simulink model "Simulation"  (R2022b)
settings: Solver=FixedStepAuto  StartTime=0.0  StopTime=param.Tsim  FixedStep=param.tSample  RelTol=1e-3
StopFcn:
  | run animation
  | run plotSol
undefined symbols (not defined in the file or in its folder): f, filterFr, filterFw, filterMr, FR_neg, FR_pos, g1, g2, g3, kFr, ki, kiSeil, kMr, kp, kpSeil, kVSl, kVSx, MR, MRP, param, xi_0
libraries: simulink x10, spsFirstOrderFilterLib x2
(part 1 of 3)
settings Model: Creator=msdirauf  LastModifiedBy=Khaled
settings SolverCC: AlgebraicLoopSolver=TrustRegion
settings DataIOCC: LimitDataPoints=on  SaveFormat=Array  ReturnWorkspaceOutputs=off
settings OptimizationCC: ExpressionDepthLimit=2147483647  LifeSpan=inf
settings DebuggingCC: UnderspecifiedInitializationDetection=Classic  MergeDetectMultiDrivingBlocksExec=none  SolverPrmCheckMsg=warning  UnconnectedInputMsg=warning  UnconnectedOutputMsg=warning  UnconnectedLineMsg=warning  StateNameClashWarn=warning  SFUnexpectedBacktrackingDiag=warning  SFNoUnconditionalDefaultTransitionDiag=warning  SFExecutionAtInitializationDiag=none  SFMachineParentedDataDiag=warning  ArithmeticOperatorsInVariantConditions=warning
settings HardwareCC: ProdBitPerPointer=32  ProdBitPerSizeT=32  ProdBitPerPtrDiffT=32  ProdLargestAtomicFloat=None  ProdIntDivRoundTo=Undefined  ProdEndianess=Unspecified  ProdWordSize=32  ProdHWDeviceType=32-bit Generic
settings ModelReferenceCC: EnableRefExpFcnMdlSchedulingChecks=on  PropagateSignalLabelsOutOfModel=off
settings SFSimCC: SimUseLocalCustomCode=off  CustomCodeUndefinedFunction=UseInterfaceOnly
settings RTWCC: RTWUseLocalCustomCode=off
settings CodeAppCC: StateflowObjectComments=on
settings GRTTargetCC: TargetLangStandard=C89/C90 (ANSI)
settings ConfigComp: CovMetricSettings=dw  CovSaveCumulativeToWorkspaceVar=on  CovSaveSingleToWorkspaceVar=on  CovExternalEMLEnable=off

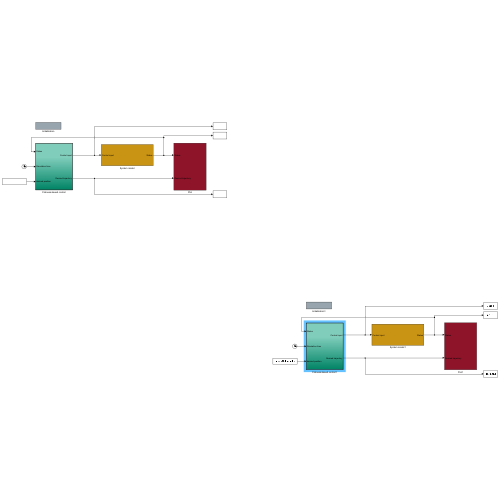
[thumbnail: Simulink's stored preview of the top-level diagram]
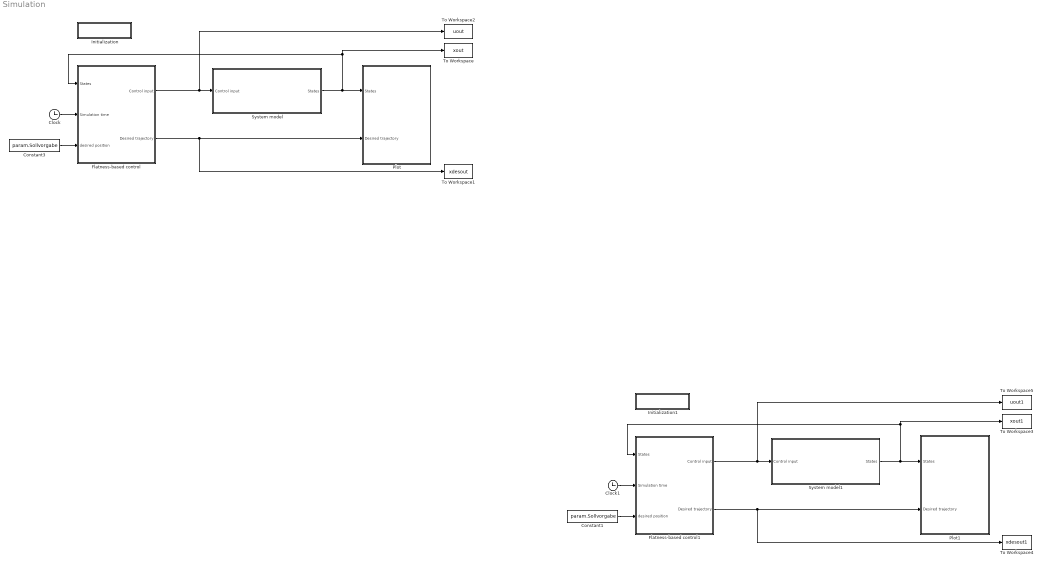
== system Simulation ==
  Clock : Clock
  Clock1 : Clock
  Constant1 : Constant  Value=param.Sollvorgabe
  Constant3 : Constant  Value=param.Sollvorgabe
  Flatness-based control : Subsystem  TreatAsAtomicUnit=on
  Flatness-based control1 : Subsystem  TreatAsAtomicUnit=on
  Initialization : Subsystem
      settings: OpenFcn=run Initialisierung_Simulation
  Initialization1 : Subsystem
      settings: OpenFcn=run Initialisierung_Simulation
  Plot : Subsystem
  Plot1 : Subsystem
  System model : Subsystem
  System model1 : Subsystem
  To Workspace : ToWorkspace  VariableName=xout  SaveFormat=Timeseries  SampleTime=-1
  To Workspace1 : ToWorkspace  VariableName=xdesout  SaveFormat=Timeseries  SampleTime=-1
  To Workspace2 : ToWorkspace  VariableName=uout  SaveFormat=Timeseries  SampleTime=-1
  To Workspace3 : ToWorkspace  VariableName=xout1  SaveFormat=Timeseries  SampleTime=-1
  To Workspace4 : ToWorkspace  VariableName=xdesout1  SaveFormat=Timeseries  SampleTime=-1
  To Workspace5 : ToWorkspace  VariableName=uout1  SaveFormat=Timeseries  SampleTime=-1
  wires:
  Flatness-based control/2(Desired trajectory) -> To Workspace1/1, Plot/2(Desired trajectory)
  Flatness-based control/1(Control input) -> To Workspace2/1, System model/1(Control input)
  Clock/1 -> Flatness-based control/2("Simulation time ")
  Constant3/1 -> Flatness-based control/3(desired position)
  System model/1(States) -> To Workspace/1, Flatness-based control/1(States), Plot/1(States)
  Flatness-based control1/2(Desired trajectory) -> To Workspace4/1, Plot1/2(Desired trajectory)
  Flatness-based control1/1(Control input) -> To Workspace5/1, System model1/1(Control input)
  Clock1/1 -> Flatness-based control1/2("Simulation time ")
  Constant1/1 -> Flatness-based control1/3(desired position)
  System model1/1(States) -> To Workspace3/1, Flatness-based control1/1(States), Plot1/1(States)

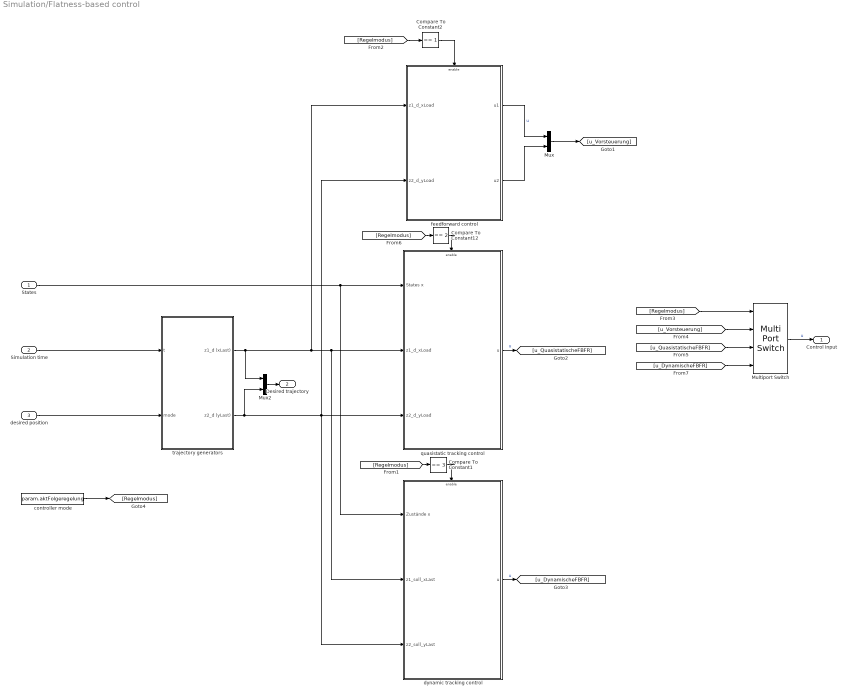
== system Simulation/Flatness-based control ==
  States : Inport
  "Simulation time " : Inport  Port=2
  desired position : Inport  Port=3
  Compare To Constant1 : simulink/Logic and Bit Operations/Compare To Constant  relop===  const=3  OutDataTypeStr=boolean  ZeroCross=off
  Compare To Constant12 : simulink/Logic and Bit Operations/Compare To Constant  relop===  const=2  OutDataTypeStr=boolean  ZeroCross=off
  Compare To Constant2 : simulink/Logic and Bit Operations/Compare To Constant  relop===  const=1  OutDataTypeStr=boolean  ZeroCross=off
  Multiport Switch : MultiPortSwitch  SaturateOnIntegerOverflow=off  InputSameDT=off
  Mux : Mux  Inputs=2
  Mux2 : Mux  Inputs=2
  controller mode : Constant  Value=param.aktFolgeregelung
  dynamic tracking control : Subsystem
  feedforward control : Subsystem
  quasistatic tracking control : Subsystem
  trajectory generators : Subsystem
  Control input : Outport  VectorParamsAs1DForOutWhenUnconnected=off
  Desired trajectory : Outport  Port=2  VectorParamsAs1DForOutWhenUnconnected=off
  wires:
  "Simulation time "/1 -> trajectory generators/1(t)
  trajectory generators/1(z1_d (xLast)) -> Mux2/1, feedforward control/1(z1_d_xLoad), quasistatic tracking control/2(z1_d_xLoad), dynamic tracking control/2(z1_soll_xLast)
  trajectory generators/2(z2_d (yLast)) -> Mux2/2, feedforward control/2(z2_d_yLoad), quasistatic tracking control/3(z2_d_yLoad), dynamic tracking control/3(z2_soll_yLast)
  desired position/1 -> trajectory generators/2(mode)
  Mux2/1 -> Desired trajectory/1
  States/1 -> quasistatic tracking control/1(States x), dynamic tracking control/1(Zustände x)
  Multiport Switch/1 -> Control input/1  "u"
  [Regelmodus] -> Multiport Switch/1
  quasistatic tracking control/1(u) -> [u_QuasistatischeFBFR]  "u"
  [u_QuasistatischeFBFR] -> Multiport Switch/3
  [u_DynamischeFBFR] -> Multiport Switch/4
  [u_Vorsteuerung] -> Multiport Switch/2
  dynamic tracking control/1(u) -> [u_DynamischeFBFR]  "u"
  controller mode/1 -> [Regelmodus]
  Compare To Constant2/1 -> feedforward control/Enable
  [Regelmodus] -> Compare To Constant2/1
  Compare To Constant12/1 -> quasistatic tracking control/Enable
  [Regelmodus] -> Compare To Constant12/1
  [Regelmodus] -> Compare To Constant1/1
  Compare To Constant1/1 -> dynamic tracking control/Enable
  feedforward control/1(u1) -> Mux/1  "u"
  Mux/1 -> [u_Vorsteuerung]
  feedforward control/2(u2) -> Mux/2

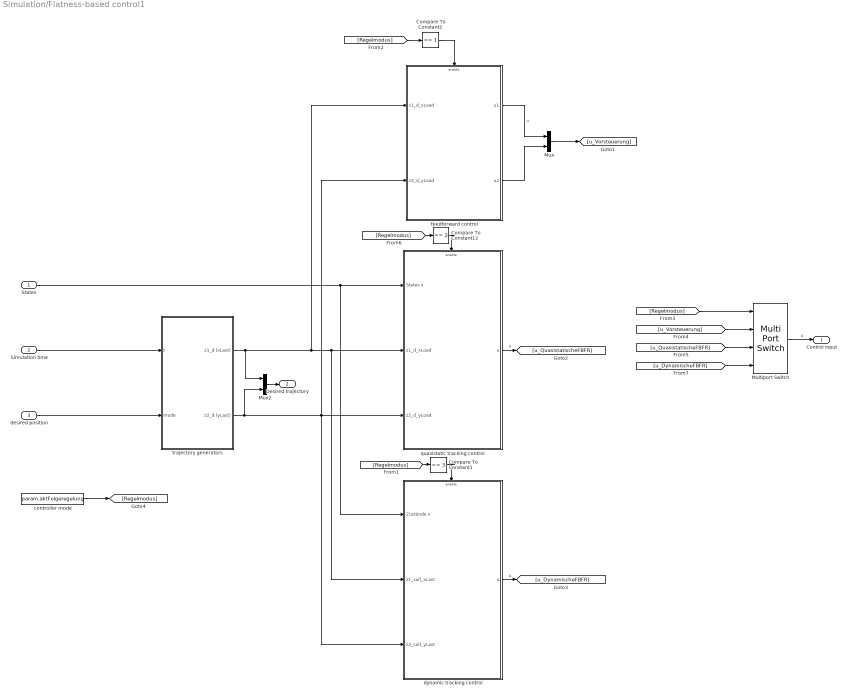
== system Simulation/Flatness-based control1 ==
  States : Inport
  "Simulation time " : Inport  Port=2
  desired position : Inport  Port=3
  Compare To Constant1 : simulink/Logic and Bit Operations/Compare To Constant  relop===  const=3  OutDataTypeStr=boolean  ZeroCross=off
  Compare To Constant12 : simulink/Logic and Bit Operations/Compare To Constant  relop===  const=2  OutDataTypeStr=boolean  ZeroCross=off
  Compare To Constant2 : simulink/Logic and Bit Operations/Compare To Constant  relop===  const=1  OutDataTypeStr=boolean  ZeroCross=off
  Multiport Switch : MultiPortSwitch  SaturateOnIntegerOverflow=off  InputSameDT=off
  Mux : Mux  Inputs=2
  Mux2 : Mux  Inputs=2
  controller mode : Constant  Value=param.aktFolgeregelung
  dynamic tracking control : Subsystem
  feedforward control : Subsystem
  quasistatic tracking control : Subsystem
  trajectory generators : Subsystem
  Control input : Outport  VectorParamsAs1DForOutWhenUnconnected=off
  Desired trajectory : Outport  Port=2  VectorParamsAs1DForOutWhenUnconnected=off
  wires:
  "Simulation time "/1 -> trajectory generators/1(t)
  trajectory generators/1(z1_d (xLast)) -> Mux2/1, feedforward control/1(z1_d_xLoad), quasistatic tracking control/2(z1_d_xLoad), dynamic tracking control/2(z1_soll_xLast)
  trajectory generators/2(z2_d (yLast)) -> Mux2/2, feedforward control/2(z2_d_yLoad), quasistatic tracking control/3(z2_d_yLoad), dynamic tracking control/3(z2_soll_yLast)
  desired position/1 -> trajectory generators/2(mode)
  Mux2/1 -> Desired trajectory/1
  States/1 -> quasistatic tracking control/1(States x), dynamic tracking control/1(Zustände x)
  Multiport Switch/1 -> Control input/1  "u"
  [Regelmodus] -> Multiport Switch/1
  quasistatic tracking control/1(u) -> [u_QuasistatischeFBFR]  "u"
  [u_QuasistatischeFBFR] -> Multiport Switch/3
  [u_DynamischeFBFR] -> Multiport Switch/4
  [u_Vorsteuerung] -> Multiport Switch/2
  dynamic tracking control/1(u) -> [u_DynamischeFBFR]  "u"
  controller mode/1 -> [Regelmodus]
  Compare To Constant2/1 -> feedforward control/Enable
  [Regelmodus] -> Compare To Constant2/1
  Compare To Constant12/1 -> quasistatic tracking control/Enable
  [Regelmodus] -> Compare To Constant12/1
  [Regelmodus] -> Compare To Constant1/1
  Compare To Constant1/1 -> dynamic tracking control/Enable
  feedforward control/1(u1) -> Mux/1  "u"
  Mux/1 -> [u_Vorsteuerung]
  feedforward control/2(u2) -> Mux/2

== system Simulation/Initialization ==

== system Simulation/Initialization1 ==

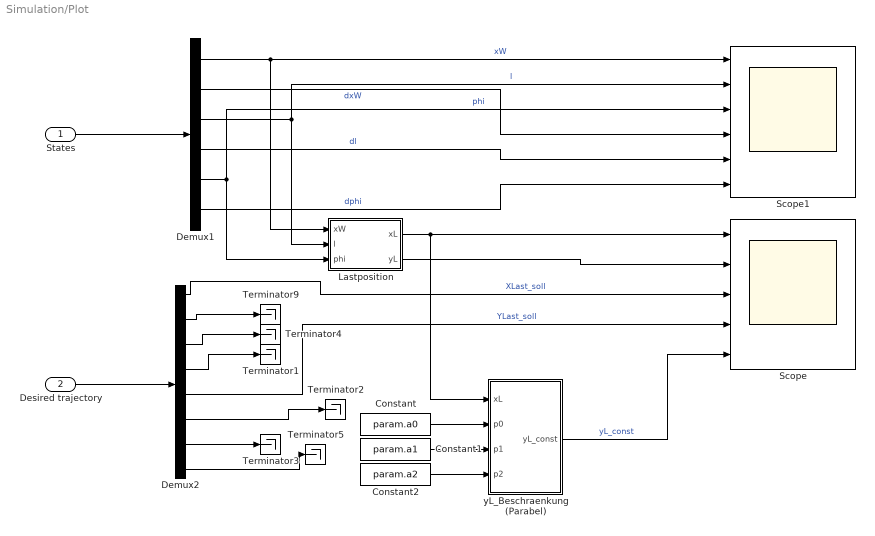
== system Simulation/Plot ==
  States : Inport
  Desired trajectory : Inport  Port=2
  Constant : Constant  Value=param.a0
  Constant1 : Constant  Value=param.a1
  Constant2 : Constant  Value=param.a2
  Demux1 : Demux  Outputs=6
  Demux2 : Demux  Outputs=8
  Lastposition : MATLAB Function  TreatAsAtomicUnit=on
  Scope : Scope  NumInputPorts=5
  Scope1 : Scope  NumInputPorts=6
  Terminator{1..5,9} (6 alike) : Terminator
  yL_Beschraenkung (Parabel) : MATLAB Function  TreatAsAtomicUnit=on
  wires:
  States/1 -> Demux1/1
  Desired trajectory/1 -> Demux2/1
  Demux2/1 -> Scope/3  "XLast_soll"
  Demux2/5 -> Scope/4  "YLast_soll"
  yL_Beschraenkung (Parabel)/1(yL_const) -> Scope/5  "yL_const"
  Demux1/1 -> Lastposition/1(xW), Scope1/1  "xW"
  Lastposition/1(xL) -> yL_Beschraenkung (Parabel)/1(xL), Scope/1
  Lastposition/2(yL) -> Scope/2
  Demux1/3 -> Lastposition/2(l), Scope1/2  "l"
  Demux1/5 -> Lastposition/3(phi), Scope1/3  "phi"
  Demux1/2 -> Scope1/4  "dxW"
  Demux1/4 -> Scope1/5  "dl"
  Demux1/6 -> Scope1/6  "dphi"
  Constant/1 -> yL_Beschraenkung (Parabel)/2(p0)
  Constant1/1 -> yL_Beschraenkung (Parabel)/3(p1)
  Demux2/2 -> Terminator9/1
  Demux2/4 -> Terminator1/1
  Demux2/6 -> Terminator2/1
  Constant2/1 -> yL_Beschraenkung (Parabel)/4(p2)
  Demux2/3 -> Terminator4/1
  Demux2/7 -> Terminator3/1
  Demux2/8 -> Terminator5/1

== system Simulation/Plot1 ==
  States : Inport
  Desired trajectory : Inport  Port=2
  Constant : Constant  Value=param.a0
  Constant1 : Constant  Value=param.a1
  Constant2 : Constant  Value=param.a2
  Demux1 : Demux  Outputs=6
  Demux2 : Demux  Outputs=8
  Lastposition : MATLAB Function  TreatAsAtomicUnit=on
  Scope : Scope  NumInputPorts=5
  Scope1 : Scope  NumInputPorts=6
  Terminator{1..5,9} (6 alike) : Terminator
  yL_Beschraenkung (Parabel) : MATLAB Function  TreatAsAtomicUnit=on
  wires:
  States/1 -> Demux1/1
  Desired trajectory/1 -> Demux2/1
  Demux2/1 -> Scope/3  "XLast_soll"
  Demux2/5 -> Scope/4  "YLast_soll"
  yL_Beschraenkung (Parabel)/1(yL_const) -> Scope/5  "yL_const"
  Demux1/1 -> Lastposition/1(xW), Scope1/1  "xW"
  Lastposition/1(xL) -> yL_Beschraenkung (Parabel)/1(xL), Scope/1
  Lastposition/2(yL) -> Scope/2
  Demux1/3 -> Lastposition/2(l), Scope1/2  "l"
  Demux1/5 -> Lastposition/3(phi), Scope1/3  "phi"
  Demux1/2 -> Scope1/4  "dxW"
  Demux1/4 -> Scope1/5  "dl"
  Demux1/6 -> Scope1/6  "dphi"
  Constant/1 -> yL_Beschraenkung (Parabel)/2(p0)
  Constant1/1 -> yL_Beschraenkung (Parabel)/3(p1)
  Demux2/2 -> Terminator9/1
  Demux2/4 -> Terminator1/1
  Demux2/6 -> Terminator2/1
  Constant2/1 -> yL_Beschraenkung (Parabel)/4(p2)
  Demux2/3 -> Terminator4/1
  Demux2/7 -> Terminator3/1
  Demux2/8 -> Terminator5/1

== system Simulation/System model ==
  Control input : Inport
  Compare To Constant : simulink/Logic and Bit Operations/Compare To Constant  relop===  const=1  OutDataTypeStr=boolean
  Compare To Constant1 : simulink/Logic and Bit Operations/Compare To Constant  relop===  const=0  OutDataTypeStr=boolean
  Constant : Constant  Value=param.Simulationsmodell
  Constant1 : Constant  Value=param.Simulationsmodell
  Constant2 : Constant  Value=param.Simulationsmodell
  Kinematisches Modell : Subsystem
  Referenzmodell : Subsystem  InitFcn=|
      | % Reglerverstaerkungen unterlagerter v-Regler Wagen
      | kp = 25; % 100
      | ki = 0;   % 0 % -> M. Lukassek: Integralanteil nicht nötig, wenn überlagert die flachheitsbasierte Folgeregelung die Sollgrößen adaptiert
      | 
      | % Reglerverstaerkungen unterlagerter v-Regler Seil
      | kpSeil = -20; % -5
      | kiSeil = -0; % -50 -> M. Lukassek: Integralanteil nicht nötig, wenn überlagert die flachheitsbasierte Folgeregelung die Sollgrößen adaptiert
      | 20
      | % Faktor Reibaufschaltung Wagen
      | kFr = 1.0;
      | filterFr = 0.1; % Zeitkonstante der Reibaufschaltung (verhindert hochfreq. Schwingen)
      | 
      | % Faktor Reibaufschaltung Seil
      | kMr = 1.0;
      | filterMr = 0.1; % Zeitkonstante der Reibaufschaltung (verhindert hochfreq. Schwingen)
      |   
      | % Stellgroesse ueberlagerte Regelung verwenden
      | kVSx = 0;  % -> M. Lukassek: Stellgrößen der FBFR als Vorsteuerung für die unterlagerte Regelung. Bypasst die Dead-Band-Reibkompensation
      | kVSl  = 0; % -> M. Lukassek: Stellgrößen der FBFR als Vorsteuerung für die unterlagerte Regelung. Bypasst die Dead-Band-Reibkompensation
      | 
      | % Filterung der Sollkraft Wagen
      | filterFw = 0;
      | filterFwT = 50e-4;
      | 
      | %% Systemparameter
      | g=9.81;
      | 
      | m1=1.43;
      | m2=0.35;
      | J=0.012477;
      | rho=0.03;
      | 
      | muVP=0.0076;
      | F_Tp=0.027;
      | F_Hp=0.012;
      | beta_P=0.073;
      | 
      | muT=0.0097;
      | c_TT=0.6;
      | c_HT=0.41;
      | omega_0=0.015;
      | 
      | mu_W_pos=2.9;
      | c_TW_pos=4.8;
      | c_HW_pos=5.7;
      | v_0_pos=0.032;
      | 
      | mu_W_neg=3.0;
      | c_TW_neg=3.9;
      | c_HW_neg=4.9;
      | v_0_neg=0.022;
      | 
      | muW=0.5*(mu_W_pos+mu_W_neg);
      | 
      | MLast=m2*g*rho;
      | 
      | % Reibparameter des Wagens (positive und negative Bewegungsrichtung)
      | param.mu_W_pos=2.9194;
      | param.c_TW_pos=4.8;
      | param.c_HW_pos=5.7;
      | param.v_0_pos=0.032;
      | 
      | param.mu_W_neg=3.0754;
      | param.c_TW_neg=3.9;
      | param.c_HW_neg=4.9;
      | param.v_0_neg=0.022;
      | 
      | param.muW=0.5*(param.mu_W_pos+param.mu_W_neg);
      | 
      | 
      | % Reibparameter der Trommel
      | param.mu_T=0.0097254;
      | param.c_TT=0.6;
      | param.c_HT=0.41;
      | param.omega_0=0.015;
      | 
      | 
      | param.MLast=param.m2*param.g*param.rho;
      | 
      | % Maximale Antriebskraft des Wagens, maximales Moment des Trommelmotors
      | param.Fmax = 22.5;  
      | param.ScaleFmax = 0.95;
      | 
      | param.M_Tmax = 3.75*rho*13; 
      | 
      | 
      | %Reibmodelle
      | MRP=@(u) u(5)*(muVP*u(2)+F_Tp*sign(u(2))+(F_Hp-F_Tp)*sign(u(2))*exp(-beta_P*abs(u(2))));
      | % ACHTUNG: es ist unklar, ob diese Gleichungen von Hand eingegeben oder
      | % oder automatisch generiert wurden. Falls letzteres, muss in der MAPLE-Quelle
      | % "rho*omega_0" durch "rho/omega_0" ersetzt werden. Hier im Matlabcode
      | % wurde das schon korrigiert.
      | MR=@(u) -(muT*u(6)/rho+c_TT*sign(u(6))+(c_HT-c_TT)*sign(u(6))*exp(-(u(6)/rho/omega_0)^2));
      | FR_pos=@(u) (mu_W_pos*u(4)+c_TW_pos*sign(u(4))+(c_HW_pos-c_TW_pos)*sign(u(4))*exp(-(u(4)/v_0_pos)^2));
      | FR_neg=@(u) (mu_W_neg*u(4)+c_TW_neg*sign(u(4))+(c_HW_neg-c_TW_neg)*sign(u(4))*exp(-(u(4)/v_0_neg)^2));
      | 
      | 
      | %% Maple-Import
      | f=@(u)  [u(2); ((2 * m2 ^ 3 * u(5) * u(2) * u(6) * rho ^ 2) + (2 * m2 ^ 2 * u(5) * u(2) * u(6) * J) + (m2 ^ 3) * g * u(5) * sin(u(1)) * (rho ^ 2) + (m2 ^ 2) * g * u(5) * sin(u(1)) * J - (m2 ^ 3) * g * u(5) * sin(u(1)) ^ 3 * (rho ^ 2) + (m2 ^ 2) * g * u(5) * sin(u(1)) * m1 * (rho ^ 2) + m2 * g * u(5) * sin(u(1)) * m1 * J + (m2 ^ 2) * cos(u(1)) * sin(u(1)) * (u(2) ^ 2) * (u(5) ^ 2) * J - 0.2e1 * (m2 ^ 3) * u(5) * u(2) * u(6) * cos(u(1)) ^ 2 * (rho ^ 2) - 0.2e1 * (m2 ^ 2) * u(5) * u(2) * u(6) * cos(u(1)) ^ 2 * J - 0.2e1 * (m2 ^ 3) * u(5) * u(2) * u(6) * sin(u(1)) ^ 2 * (rho ^ 2) - (m2 ^ 3) * g * u(5) * sin(u(1)) * cos(u(1)) ^ 2 * (rho ^ 2) + 0.2e1 * (m2 ^ 2) * u(5) * u(2) * u(6) * m1 * (rho ^ 2) + 0.2e1 * m2 * u(5) * u(2) * u(6) * m1 * J) / (u(5) ^ 2) / ((m2 ^ 2) * cos(u(1)) ^ 2 * (rho ^ 2) + m2 * cos(u(1)) ^ 2 * J - m1 * m2 * (rho ^ 2) - m1 * J - (m2 ^ 2 * rho ^ 2) - (m2 * J) + (m2 ^ 2) * sin(u(1)) ^ 2 * (rho ^ 2)) / m2; u(4); -0.1e1 / ((m2 ^ 2) * cos(u(1)) ^ 2 * (rho ^ 2) + m2 * cos(u(1)) ^ 2 * J - m1 * m2 * (rho ^ 2) - m1 * J - (m2 ^ 2 * rho ^ 2) - (m2 * J) + (m2 ^ 2) * sin(u(1)) ^ 2 * (rho ^ 2)) * (cos(u(1)) * m2 * g * u(5) * sin(u(1)) * J + m2 * sin(u(1)) * (u(2) ^ 2) * (u(5) ^ 2) * J) / u(5); u(6); ((m2 ^ 2) * sin(u(1)) ^ 2 * rho * cos(u(1)) * g * u(5) - u(5) * m2 * g * cos(u(1)) * rho * m1 - (m2 ^ 2 * u(5) ^ 2 * u(2) ^ 2 * rho) + (m2 ^ 2) * sin(u(1)) ^ 2 * rho * (u(2) ^ 2) * (u(5) ^ 2) + u(5) * (m2 ^ 2) * g * cos(u(1)) ^ 3 * rho - u(5) * (m2 ^ 2) * g * cos(u(1)) * rho + (m2 ^ 2) * (u(5) ^ 2) * (u(2) ^ 2) * rho * cos(u(1)) ^ 2 - m2 * (u(5) ^ 2) * (u(2) ^ 2) * rho * m1) * rho / ((m2 ^ 2) * cos(u(1)) ^ 2 * (rho ^ 2) + m2 * cos(u(1)) ^ 2 * J - m1 * m2 * (rho ^ 2) - m1 * J - (m2 ^ 2 * rho ^ 2) - (m2 * J) + (m2 ^ 2) * sin(u(1)) ^ 2 * (rho ^ 2)) / u(5);];
      | g1=@(u) [0; cos(u(1)) * (m2 * rho ^ 2 + J) / (m2 * cos(u(1)) ^ 2 * J - m2 * J - m1 * m2 * rho ^ 2 - m1 * J) / u(5); 0; -(m2 * rho ^ 2 + J) / (m2 * cos(u(1)) ^ 2 * J - m2 * J - m1 * m2 * rho ^ 2 - m1 * J); 0; m2 * sin(u(1)) * rho ^ 2 / (m2 * cos(u(1)) ^ 2 * J - m2 * J - m1 * m2 * rho ^ 2 - m1 * J);];
      | g2=@(u) [0; m2 * cos(u(1)) * sin(u(1)) * rho / (m2 * cos(u(1)) ^ 2 * J - m2 * J - m1 * m2 * rho ^ 2 - m1 * J) / u(5); 0; -m2 * sin(u(1)) * rho / (m2 * cos(u(1)) ^ 2 * J - m2 * J - m1 * m2 * rho ^ 2 - m1 * J); 0; -rho * (m2 * cos(u(1)) ^ 2 - m1 - m2) / (m2 * cos(u(1)) ^ 2 * J - m2 * J - m1 * m2 * rho ^ 2 - m1 * J);];
      | g3=@(u) [0; (m2 * J + m1 * m2 * rho ^ 2 + m1 * J + m2 ^ 2 * cos(u(1)) ^ 2 * rho ^ 2) / (m2 * cos(u(1)) ^ 2 * J - m2 * J - m1 * m2 * rho ^ 2 - m1 * J) / m2 / u(5) ^ 2; 0; -cos(u(1)) * (m2 * rho ^ 2 + J) / (m2 * cos(u(1)) ^ 2 * J - m2 * J - m1 * m2 * rho ^ 2 - m1 * J) / u(5); 0; m2 * rho ^ 2 * sin(u(1)) * cos(u(1)) / (m2 * cos(u(1)) ^ 2 * J - m2 * J - m1 * m2 * rho ^ 2 - m1 * J) / u(5);];
  Switch : Switch  Criteria=u2 > Threshold  SaturateOnIntegerOverflow=off  InputSameDT=off
  States : Outport  VectorParamsAs1DForOutWhenUnconnected=off
  wires:
  Control input/1 -> Referenzmodell/1(Stellgroessen), Kinematisches Modell/1(Stellgroessen)
  Switch/1 -> States/1
  Kinematisches Modell/1(Systemzustände) -> Switch/3
  Referenzmodell/1(Systemzustaende) -> Switch/1
  Constant/1 -> Switch/2
  Constant1/1 -> Compare To Constant/1
  Compare To Constant/1 -> Referenzmodell/Enable
  Constant2/1 -> Compare To Constant1/1
  Compare To Constant1/1 -> Kinematisches Modell/Enable

== system Simulation/System model1 ==
  Control input : Inport
  Compare To Constant : simulink/Logic and Bit Operations/Compare To Constant  relop===  const=1  OutDataTypeStr=boolean
  Compare To Constant1 : simulink/Logic and Bit Operations/Compare To Constant  relop===  const=0  OutDataTypeStr=boolean
  Constant : Constant  Value=param.Simulationsmodell
  Constant1 : Constant  Value=param.Simulationsmodell
  Constant2 : Constant  Value=param.Simulationsmodell
  Kinematisches Modell : Subsystem
  Referenzmodell : Subsystem  InitFcn=|
      | % Reglerverstaerkungen unterlagerter v-Regler Wagen
      | kp = 25; % 100
      | ki = 0;   % 0 % -> M. Lukassek: Integralanteil nicht nötig, wenn überlagert die flachheitsbasierte Folgeregelung die Sollgrößen adaptiert
      | 
      | % Reglerverstaerkungen unterlagerter v-Regler Seil
      | kpSeil = -20; % -5
      | kiSeil = -0; % -50 -> M. Lukassek: Integralanteil nicht nötig, wenn überlagert die flachheitsbasierte Folgeregelung die Sollgrößen adaptiert
      | 20
      | % Faktor Reibaufschaltung Wagen
      | kFr = 1.0;
      | filterFr = 0.1; % Zeitkonstante der Reibaufschaltung (verhindert hochfreq. Schwingen)
      | 
      | % Faktor Reibaufschaltung Seil
      | kMr = 1.0;
      | filterMr = 0.1; % Zeitkonstante der Reibaufschaltung (verhindert hochfreq. Schwingen)
      |   
      | % Stellgroesse ueberlagerte Regelung verwenden
      | kVSx = 0;  % -> M. Lukassek: Stellgrößen der FBFR als Vorsteuerung für die unterlagerte Regelung. Bypasst die Dead-Band-Reibkompensation
      | kVSl  = 0; % -> M. Lukassek: Stellgrößen der FBFR als Vorsteuerung für die unterlagerte Regelung. Bypasst die Dead-Band-Reibkompensation
      | 
      | % Filterung der Sollkraft Wagen
      | filterFw = 0;
      | filterFwT = 50e-4;
      | 
      | %% Systemparameter
      | g=9.81;
      | 
      | m1=1.43;
      | m2=0.35;
      | J=0.012477;
      | rho=0.03;
      | 
      | muVP=0.0076;
      | F_Tp=0.027;
      | F_Hp=0.012;
      | beta_P=0.073;
      | 
      | muT=0.0097;
      | c_TT=0.6;
      | c_HT=0.41;
      | omega_0=0.015;
      | 
      | mu_W_pos=2.9;
      | c_TW_pos=4.8;
      | c_HW_pos=5.7;
      | v_0_pos=0.032;
      | 
      | mu_W_neg=3.0;
      | c_TW_neg=3.9;
      | c_HW_neg=4.9;
      | v_0_neg=0.022;
      | 
      | muW=0.5*(mu_W_pos+mu_W_neg);
      | 
      | MLast=m2*g*rho;
      | 
      | % Reibparameter des Wagens (positive und negative Bewegungsrichtung)
      | param.mu_W_pos=2.9194;
      | param.c_TW_pos=4.8;
      | param.c_HW_pos=5.7;
      | param.v_0_pos=0.032;
      | 
      | param.mu_W_neg=3.0754;
      | param.c_TW_neg=3.9;
      | param.c_HW_neg=4.9;
      | param.v_0_neg=0.022;
      | 
      | param.muW=0.5*(param.mu_W_pos+param.mu_W_neg);
      | 
      | 
      | % Reibparameter der Trommel
      | param.mu_T=0.0097254;
      | param.c_TT=0.6;
      | param.c_HT=0.41;
      | param.omega_0=0.015;
      | 
      | 
      | param.MLast=param.m2*param.g*param.rho;
      | 
      | % Maximale Antriebskraft des Wagens, maximales Moment des Trommelmotors
      | param.Fmax = 22.5;  
      | param.ScaleFmax = 0.95;
      | 
      | param.M_Tmax = 3.75*rho*13; 
      | 
      | 
      | %Reibmodelle
      | MRP=@(u) u(5)*(muVP*u(2)+F_Tp*sign(u(2))+(F_Hp-F_Tp)*sign(u(2))*exp(-beta_P*abs(u(2))));
      | % ACHTUNG: es ist unklar, ob diese Gleichungen von Hand eingegeben oder
      | % oder automatisch generiert wurden. Falls letzteres, muss in der MAPLE-Quelle
      | % "rho*omega_0" durch "rho/omega_0" ersetzt werden. Hier im Matlabcode
      | % wurde das schon korrigiert.
      | MR=@(u) -(muT*u(6)/rho+c_TT*sign(u(6))+(c_HT-c_TT)*sign(u(6))*exp(-(u(6)/rho/omega_0)^2));
      | FR_pos=@(u) (mu_W_pos*u(4)+c_TW_pos*sign(u(4))+(c_HW_pos-c_TW_pos)*sign(u(4))*exp(-(u(4)/v_0_pos)^2));
      | FR_neg=@(u) (mu_W_neg*u(4)+c_TW_neg*sign(u(4))+(c_HW_neg-c_TW_neg)*sign(u(4))*exp(-(u(4)/v_0_neg)^2));
      | 
      | 
      | %% Maple-Import
      | f=@(u)  [u(2); ((2 * m2 ^ 3 * u(5) * u(2) * u(6) * rho ^ 2) + (2 * m2 ^ 2 * u(5) * u(2) * u(6) * J) + (m2 ^ 3) * g * u(5) * sin(u(1)) * (rho ^ 2) + (m2 ^ 2) * g * u(5) * sin(u(1)) * J - (m2 ^ 3) * g * u(5) * sin(u(1)) ^ 3 * (rho ^ 2) + (m2 ^ 2) * g * u(5) * sin(u(1)) * m1 * (rho ^ 2) + m2 * g * u(5) * sin(u(1)) * m1 * J + (m2 ^ 2) * cos(u(1)) * sin(u(1)) * (u(2) ^ 2) * (u(5) ^ 2) * J - 0.2e1 * (m2 ^ 3) * u(5) * u(2) * u(6) * cos(u(1)) ^ 2 * (rho ^ 2) - 0.2e1 * (m2 ^ 2) * u(5) * u(2) * u(6) * cos(u(1)) ^ 2 * J - 0.2e1 * (m2 ^ 3) * u(5) * u(2) * u(6) * sin(u(1)) ^ 2 * (rho ^ 2) - (m2 ^ 3) * g * u(5) * sin(u(1)) * cos(u(1)) ^ 2 * (rho ^ 2) + 0.2e1 * (m2 ^ 2) * u(5) * u(2) * u(6) * m1 * (rho ^ 2) + 0.2e1 * m2 * u(5) * u(2) * u(6) * m1 * J) / (u(5) ^ 2) / ((m2 ^ 2) * cos(u(1)) ^ 2 * (rho ^ 2) + m2 * cos(u(1)) ^ 2 * J - m1 * m2 * (rho ^ 2) - m1 * J - (m2 ^ 2 * rho ^ 2) - (m2 * J) + (m2 ^ 2) * sin(u(1)) ^ 2 * (rho ^ 2)) / m2; u(4); -0.1e1 / ((m2 ^ 2) * cos(u(1)) ^ 2 * (rho ^ 2) + m2 * cos(u(1)) ^ 2 * J - m1 * m2 * (rho ^ 2) - m1 * J - (m2 ^ 2 * rho ^ 2) - (m2 * J) + (m2 ^ 2) * sin(u(1)) ^ 2 * (rho ^ 2)) * (cos(u(1)) * m2 * g * u(5) * sin(u(1)) * J + m2 * sin(u(1)) * (u(2) ^ 2) * (u(5) ^ 2) * J) / u(5); u(6); ((m2 ^ 2) * sin(u(1)) ^ 2 * rho * cos(u(1)) * g * u(5) - u(5) * m2 * g * cos(u(1)) * rho * m1 - (m2 ^ 2 * u(5) ^ 2 * u(2) ^ 2 * rho) + (m2 ^ 2) * sin(u(1)) ^ 2 * rho * (u(2) ^ 2) * (u(5) ^ 2) + u(5) * (m2 ^ 2) * g * cos(u(1)) ^ 3 * rho - u(5) * (m2 ^ 2) * g * cos(u(1)) * rho + (m2 ^ 2) * (u(5) ^ 2) * (u(2) ^ 2) * rho * cos(u(1)) ^ 2 - m2 * (u(5) ^ 2) * (u(2) ^ 2) * rho * m1) * rho / ((m2 ^ 2) * cos(u(1)) ^ 2 * (rho ^ 2) + m2 * cos(u(1)) ^ 2 * J - m1 * m2 * (rho ^ 2) - m1 * J - (m2 ^ 2 * rho ^ 2) - (m2 * J) + (m2 ^ 2) * sin(u(1)) ^ 2 * (rho ^ 2)) / u(5);];
      | g1=@(u) [0; cos(u(1)) * (m2 * rho ^ 2 + J) / (m2 * cos(u(1)) ^ 2 * J - m2 * J - m1 * m2 * rho ^ 2 - m1 * J) / u(5); 0; -(m2 * rho ^ 2 + J) / (m2 * cos(u(1)) ^ 2 * J - m2 * J - m1 * m2 * rho ^ 2 - m1 * J); 0; m2 * sin(u(1)) * rho ^ 2 / (m2 * cos(u(1)) ^ 2 * J - m2 * J - m1 * m2 * rho ^ 2 - m1 * J);];
      | g2=@(u) [0; m2 * cos(u(1)) * sin(u(1)) * rho / (m2 * cos(u(1)) ^ 2 * J - m2 * J - m1 * m2 * rho ^ 2 - m1 * J) / u(5); 0; -m2 * sin(u(1)) * rho / (m2 * cos(u(1)) ^ 2 * J - m2 * J - m1 * m2 * rho ^ 2 - m1 * J); 0; -rho * (m2 * cos(u(1)) ^ 2 - m1 - m2) / (m2 * cos(u(1)) ^ 2 * J - m2 * J - m1 * m2 * rho ^ 2 - m1 * J);];
      | g3=@(u) [0; (m2 * J + m1 * m2 * rho ^ 2 + m1 * J + m2 ^ 2 * cos(u(1)) ^ 2 * rho ^ 2) / (m2 * cos(u(1)) ^ 2 * J - m2 * J - m1 * m2 * rho ^ 2 - m1 * J) / m2 / u(5) ^ 2; 0; -cos(u(1)) * (m2 * rho ^ 2 + J) / (m2 * cos(u(1)) ^ 2 * J - m2 * J - m1 * m2 * rho ^ 2 - m1 * J) / u(5); 0; m2 * rho ^ 2 * sin(u(1)) * cos(u(1)) / (m2 * cos(u(1)) ^ 2 * J - m2 * J - m1 * m2 * rho ^ 2 - m1 * J) / u(5);];
  Switch : Switch  Criteria=u2 > Threshold  SaturateOnIntegerOverflow=off  InputSameDT=off
  States : Outport  VectorParamsAs1DForOutWhenUnconnected=off
  wires:
  Control input/1 -> Referenzmodell/1(Stellgroessen), Kinematisches Modell/1(Stellgroessen)
  Switch/1 -> States/1
  Kinematisches Modell/1(Systemzustände) -> Switch/3
  Referenzmodell/1(Systemzustaende) -> Switch/1
  Constant/1 -> Switch/2
  Constant1/1 -> Compare To Constant/1
  Compare To Constant/1 -> Referenzmodell/Enable
  Constant2/1 -> Compare To Constant1/1
  Compare To Constant1/1 -> Kinematisches Modell/Enable

== system Simulation/Flatness-based control/dynamic tracking control ==
  Zustände x : Inport
  z1_soll_xLast : Inport  Port=2
  z2_soll_yLast : Inport  Port=3
  EnableDynamischeFBFR : EnablePort  StatesWhenEnabling=reset
  Computation of the flat output : Subsystem
  Mux1 : Mux  Inputs=2
  Mux5 : Mux  Inputs=2
  System extension : Subsystem
  Tracking controller : Subsystem
  Unit Delay1 : UnitDelay  InitialCondition=[0;0]  SampleTime=-1  HasFrameUpgradeWarning=on
  u : Outport
  wires:
  Mux5/1 -> u/1  "u_real"
  System extension/2(x_extended) -> Computation of the flat output/2(States)
  z1_soll_xLast/1 -> Tracking controller/3(z1_d_xLoad)
  Tracking controller/1(u1_aCart) -> Mux5/1, Mux1/1  "u1"
  Computation of the flat output/2(z2_yLoad) -> Tracking controller/2(z2_yLoad)
  Unit Delay1/1 -> System extension/1(u_extended), Computation of the flat output/1(Control input)  "u_old"
  z2_soll_yLast/1 -> Tracking controller/4(z2_d_yLoad)
  Tracking controller/2(u2_aRope) -> Mux1/2  "aRope_d"
  Mux1/1 -> Unit Delay1/1  "u"
  Computation of the flat output/1(z1_xLoad) -> Tracking controller/1(z1_xLoad)
  System extension/1(u2_real) -> Mux5/2  "u2_real"
  Zustände x/1 -> System extension/2(x_real)

== system Simulation/Flatness-based control/feedforward control ==
  z1_d_xLoad : Inport
  z2_d_yLoad : Inport  Port=2
  EnableFBFF : EnablePort  StatesWhenEnabling=reset
  Demux : Demux
  Demux1 : Demux
  MATLAB Function : MATLAB Function  TreatAsAtomicUnit=on
  u1 : Outport
  u2 : Outport  Port=2
  wires:
  z1_d_xLoad/1 -> Demux/1
  MATLAB Function/1(u1) -> u1/1
  MATLAB Function/2(u2) -> u2/1
  Demux/1 -> MATLAB Function/1(z1)
  Demux/2 -> MATLAB Function/2(dz1)
  Demux/3 -> MATLAB Function/3(ddz1)
  z2_d_yLoad/1 -> Demux1/1
  Demux1/1 -> MATLAB Function/5(z2)
  Demux1/2 -> MATLAB Function/6(dz2)
  Demux1/3 -> MATLAB Function/7(ddz2)
  Demux/4 -> MATLAB Function/4(d3z1)
  Demux1/4 -> MATLAB Function/8(d3z2)

== system Simulation/Flatness-based control/quasistatic tracking control ==
  States x : Inport
  z1_d_xLoad : Inport  Port=2
  z2_d_yLoad : Inport  Port=3
  EnableQuasistatischeFBFR : EnablePort  StatesWhenEnabling=reset
  Computation of the flat output : Subsystem
  Mux : Mux  Inputs=2
  Tracking controller : Subsystem
  Unit Delay : UnitDelay  InitialCondition=[0;0]  SampleTime=-1  HasFrameUpgradeWarning=on
  u : Outport
  wires:
  Computation of the flat output/2(z2_yLoad) -> Tracking controller/2(z2_yLoad)
  Computation of the flat output/1(z1_xLoad) -> Tracking controller/1(z1_xLoad)
  Tracking controller/2(u2_aRope) -> Mux/2  "aRope_d"
  Mux/1 -> u/1, Unit Delay/1  "u"
  Unit Delay/1 -> Computation of the flat output/1(Control input)  "u_old"
  States x/1 -> Computation of the flat output/2(States)
  Tracking controller/1(u1_aCart) -> Mux/1  "u1"
  z1_d_xLoad/1 -> Tracking controller/3(z1_d_xLoad)
  z2_d_yLoad/1 -> Tracking controller/4(z2_d_yLoad)

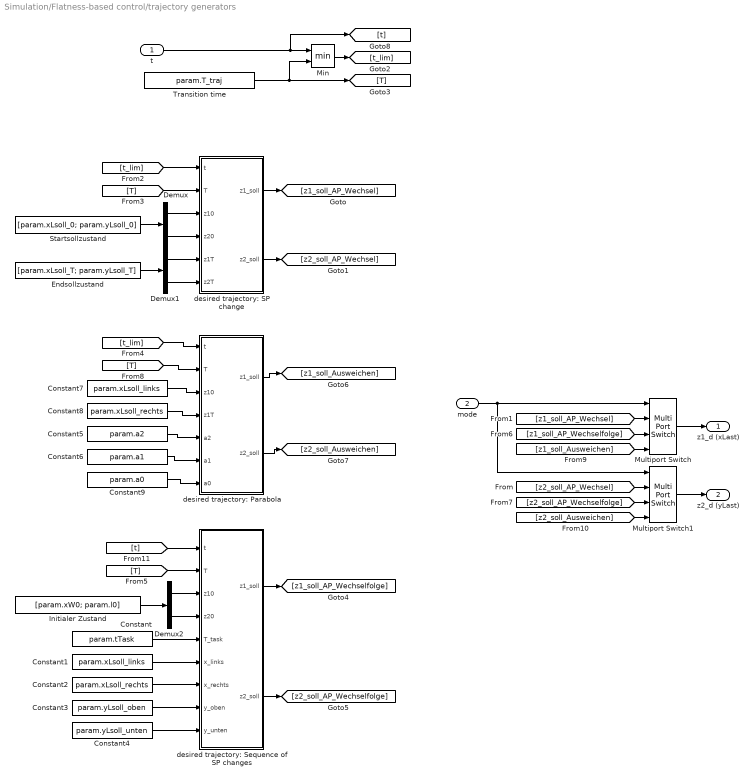
== system Simulation/Flatness-based control/trajectory generators ==
  t : Inport
  mode : Inport  Port=2
  Constant : Constant  Value=param.tTask
  Constant1 : Constant  Value=param.xLsoll_links
  Constant2 : Constant  Value=param.xLsoll_rechts
  Constant3 : Constant  Value=param.yLsoll_oben
  Constant4 : Constant  Value=param.yLsoll_unten
  Constant5 : Constant  Value=param.a2
  Constant6 : Constant  Value=param.a1
  Constant7 : Constant  Value=param.xLsoll_links
  Constant8 : Constant  Value=param.xLsoll_rechts
  Constant9 : Constant  Value=param.a0
  Demux : Demux  Outputs=2
  Demux1 : Demux  Outputs=2
  Demux2 : Demux  Outputs=2
  Endsollzustand : Constant  Value=[param.xLsoll_T; param.yLsoll_T]
  Initialer Zustand : Constant  Value=[param.xW0; param.l0]
  Min : MinMax  Inputs=2
  Multiport Switch : MultiPortSwitch  SaturateOnIntegerOverflow=off  InputSameDT=off
  Multiport Switch1 : MultiPortSwitch  SaturateOnIntegerOverflow=off  InputSameDT=off
  Startsollzustand : Constant  Value=[param.xLsoll_0; param.yLsoll_0]
  Transition time : Constant  Value=param.T_traj
  desired trajectory: Parabola : MATLAB Function  TreatAsAtomicUnit=on
  desired trajectory: SP change : MATLAB Function  TreatAsAtomicUnit=on
  desired trajectory: Sequence of SP changes : MATLAB Function  TreatAsAtomicUnit=on
  z1_d (xLast) : Outport
  z2_d (yLast) : Outport  Port=2
  wires:
  Transition time/1 -> [T], Min/2
  mode/1 -> Multiport Switch/1, Multiport Switch1/1
  Multiport Switch1/1 -> z2_d (yLast)/1
  Multiport Switch/1 -> z1_d (xLast)/1
  [z2_soll_AP_Wechsel] -> Multiport Switch1/2
  [z1_soll_AP_Wechsel] -> Multiport Switch/2
  Min/1 -> [t_lim]
  t/1 -> [t], Min/1
  [z1_soll_AP_Wechselfolge] -> Multiport Switch/3
  [z2_soll_AP_Wechselfolge] -> Multiport Switch1/3
  Startsollzustand/1 -> Demux/1
  Endsollzustand/1 -> Demux1/1
  [z1_soll_Ausweichen] -> Multiport Switch/4
  [z2_soll_Ausweichen] -> Multiport Switch1/4
  Initialer Zustand/1 -> Demux2/1
  [t_lim] -> desired trajectory: SP change/1(t)
  [T] -> desired trajectory: SP change/2(T)
  Demux/1 -> desired trajectory: SP change/3(z10)
  Demux/2 -> desired trajectory: SP change/4(z20)
  Demux1/1 -> desired trajectory: SP change/5(z1T)
  Demux1/2 -> desired trajectory: SP change/6(z2T)
  desired trajectory: SP change/1(z1_soll) -> [z1_soll_AP_Wechsel]
  desired trajectory: SP change/2(z2_soll) -> [z2_soll_AP_Wechsel]
  [t_lim] -> desired trajectory: Parabola/1(t)
  [T] -> desired trajectory: Parabola/2(T)
  Constant7/1 -> desired trajectory: Parabola/3(z10)
  Constant8/1 -> desired trajectory: Parabola/4(z1T)
  Constant5/1 -> desired trajectory: Parabola/5(a2)
  Constant6/1 -> desired trajectory: Parabola/6(a1)
  Constant9/1 -> desired trajectory: Parabola/7(a0)
  desired trajectory: Parabola/1(z1_soll) -> [z1_soll_Ausweichen]
  desired trajectory: Parabola/2(z2_soll) -> [z2_soll_Ausweichen]
  [t] -> desired trajectory: Sequence of SP changes/1(t)
  [T] -> desired trajectory: Sequence of SP changes/2(T)
  Demux2/1 -> desired trajectory: Sequence of SP changes/3(z10)
  Demux2/2 -> desired trajectory: Sequence of SP changes/4(z20)
  Constant/1 -> desired trajectory: Sequence of SP changes/5(T_task)
  Constant1/1 -> desired trajectory: Sequence of SP changes/6(x_links)
  Constant2/1 -> desired trajectory: Sequence of SP changes/7(x_rechts)
  Constant3/1 -> desired trajectory: Sequence of SP changes/8(y_oben)
  Constant4/1 -> desired trajectory: Sequence of SP changes/9(y_unten)
  desired trajectory: Sequence of SP changes/1(z1_soll) -> [z1_soll_AP_Wechselfolge]
  desired trajectory: Sequence of SP changes/2(z2_soll) -> [z2_soll_AP_Wechselfolge]

== system Simulation/Flatness-based control1/dynamic tracking control ==
  Zustände x : Inport
  z1_soll_xLast : Inport  Port=2
  z2_soll_yLast : Inport  Port=3
  EnableDynamischeFBFR : EnablePort  StatesWhenEnabling=reset
  Computation of the flat output : Subsystem
  Mux1 : Mux  Inputs=2
  Mux5 : Mux  Inputs=2
  System extension : Subsystem
  Tracking controller : Subsystem
  Unit Delay1 : UnitDelay  InitialCondition=[0;0]  SampleTime=-1  HasFrameUpgradeWarning=on
  u : Outport
  wires:
  Mux5/1 -> u/1  "u_real"
  System extension/2(x_extended) -> Computation of the flat output/2(States)
  z1_soll_xLast/1 -> Tracking controller/3(z1_d_xLoad)
  Tracking controller/1(u1_aCart) -> Mux5/1, Mux1/1  "u1"
  Computation of the flat output/2(z2_yLoad) -> Tracking controller/2(z2_yLoad)
  Unit Delay1/1 -> System extension/1(u_extended), Computation of the flat output/1(Control input)  "u_old"
  z2_soll_yLast/1 -> Tracking controller/4(z2_d_yLoad)
  Tracking controller/2(u2_aRope) -> Mux1/2  "aRope_d"
  Mux1/1 -> Unit Delay1/1  "u"
  Computation of the flat output/1(z1_xLoad) -> Tracking controller/1(z1_xLoad)
  System extension/1(u2_real) -> Mux5/2  "u2_real"
  Zustände x/1 -> System extension/2(x_real)

== system Simulation/Flatness-based control1/feedforward control ==
  z1_d_xLoad : Inport
  z2_d_yLoad : Inport  Port=2
  EnableFBFF : EnablePort  StatesWhenEnabling=reset
  Demux : Demux
  Demux1 : Demux
  MATLAB Function : MATLAB Function  TreatAsAtomicUnit=on
  u1 : Outport
  u2 : Outport  Port=2
  wires:
  z1_d_xLoad/1 -> Demux/1
  MATLAB Function/1(u1) -> u1/1
  MATLAB Function/2(u2) -> u2/1
  Demux/1 -> MATLAB Function/1(z1)
  Demux/2 -> MATLAB Function/2(dz1)
  Demux/3 -> MATLAB Function/3(ddz1)
  z2_d_yLoad/1 -> Demux1/1
  Demux1/1 -> MATLAB Function/5(z2)
  Demux1/2 -> MATLAB Function/6(dz2)
  Demux1/3 -> MATLAB Function/7(ddz2)
  Demux/4 -> MATLAB Function/4(d3z1)
  Demux1/4 -> MATLAB Function/8(d3z2)

== system Simulation/Flatness-based control1/quasistatic tracking control ==
  States x : Inport
  z1_d_xLoad : Inport  Port=2
  z2_d_yLoad : Inport  Port=3
  EnableQuasistatischeFBFR : EnablePort  StatesWhenEnabling=reset
  Computation of the flat output : Subsystem
  Mux : Mux  Inputs=2
  Tracking controller : Subsystem
  Unit Delay : UnitDelay  InitialCondition=[0;0]  SampleTime=-1  HasFrameUpgradeWarning=on
  u : Outport
  wires:
  Computation of the flat output/2(z2_yLoad) -> Tracking controller/2(z2_yLoad)
  Computation of the flat output/1(z1_xLoad) -> Tracking controller/1(z1_xLoad)
  Tracking controller/2(u2_aRope) -> Mux/2  "aRope_d"
  Mux/1 -> u/1, Unit Delay/1  "u"
  Unit Delay/1 -> Computation of the flat output/1(Control input)  "u_old"
  States x/1 -> Computation of the flat output/2(States)
  Tracking controller/1(u1_aCart) -> Mux/1  "u1"
  z1_d_xLoad/1 -> Tracking controller/3(z1_d_xLoad)
  z2_d_yLoad/1 -> Tracking controller/4(z2_d_yLoad)

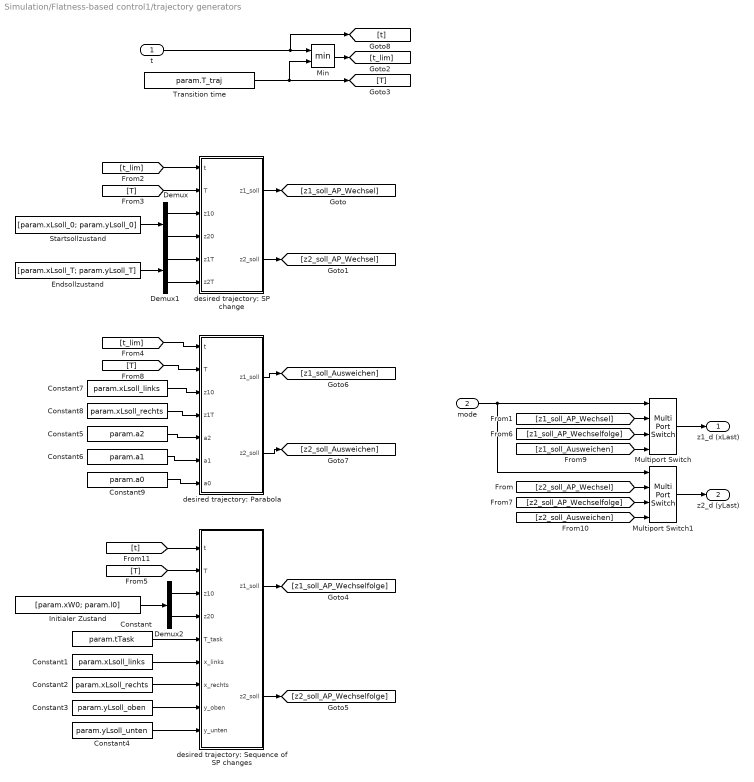
== system Simulation/Flatness-based control1/trajectory generators ==
  t : Inport
  mode : Inport  Port=2
  Constant : Constant  Value=param.tTask
  Constant1 : Constant  Value=param.xLsoll_links
  Constant2 : Constant  Value=param.xLsoll_rechts
  Constant3 : Constant  Value=param.yLsoll_oben
  Constant4 : Constant  Value=param.yLsoll_unten
  Constant5 : Constant  Value=param.a2
  Constant6 : Constant  Value=param.a1
  Constant7 : Constant  Value=param.xLsoll_links
  Constant8 : Constant  Value=param.xLsoll_rechts
  Constant9 : Constant  Value=param.a0
  Demux : Demux  Outputs=2
  Demux1 : Demux  Outputs=2
  Demux2 : Demux  Outputs=2
  Endsollzustand : Constant  Value=[param.xLsoll_T; param.yLsoll_T]
  Initialer Zustand : Constant  Value=[param.xW0; param.l0]
  Min : MinMax  Inputs=2
  Multiport Switch : MultiPortSwitch  SaturateOnIntegerOverflow=off  InputSameDT=off
  Multiport Switch1 : MultiPortSwitch  SaturateOnIntegerOverflow=off  InputSameDT=off
  Startsollzustand : Constant  Value=[param.xLsoll_0; param.yLsoll_0]
  Transition time : Constant  Value=param.T_traj
  desired trajectory: Parabola : MATLAB Function  TreatAsAtomicUnit=on
  desired trajectory: SP change : MATLAB Function  TreatAsAtomicUnit=on
  desired trajectory: Sequence of SP changes : MATLAB Function  TreatAsAtomicUnit=on
  z1_d (xLast) : Outport
  z2_d (yLast) : Outport  Port=2
  wires:
  Transition time/1 -> [T], Min/2
  mode/1 -> Multiport Switch/1, Multiport Switch1/1
  Multiport Switch1/1 -> z2_d (yLast)/1
  Multiport Switch/1 -> z1_d (xLast)/1
  [z2_soll_AP_Wechsel] -> Multiport Switch1/2
  [z1_soll_AP_Wechsel] -> Multiport Switch/2
  Min/1 -> [t_lim]
  t/1 -> [t], Min/1
  [z1_soll_AP_Wechselfolge] -> Multiport Switch/3
  [z2_soll_AP_Wechselfolge] -> Multiport Switch1/3
  Startsollzustand/1 -> Demux/1
  Endsollzustand/1 -> Demux1/1
  [z1_soll_Ausweichen] -> Multiport Switch/4
  [z2_soll_Ausweichen] -> Multiport Switch1/4
  Initialer Zustand/1 -> Demux2/1
  [t_lim] -> desired trajectory: SP change/1(t)
  [T] -> desired trajectory: SP change/2(T)
  Demux/1 -> desired trajectory: SP change/3(z10)
  Demux/2 -> desired trajectory: SP change/4(z20)
  Demux1/1 -> desired trajectory: SP change/5(z1T)
  Demux1/2 -> desired trajectory: SP change/6(z2T)
  desired trajectory: SP change/1(z1_soll) -> [z1_soll_AP_Wechsel]
  desired trajectory: SP change/2(z2_soll) -> [z2_soll_AP_Wechsel]
  [t_lim] -> desired trajectory: Parabola/1(t)
  [T] -> desired trajectory: Parabola/2(T)
  Constant7/1 -> desired trajectory: Parabola/3(z10)
  Constant8/1 -> desired trajectory: Parabola/4(z1T)
  Constant5/1 -> desired trajectory: Parabola/5(a2)
  Constant6/1 -> desired trajectory: Parabola/6(a1)
  Constant9/1 -> desired trajectory: Parabola/7(a0)
  desired trajectory: Parabola/1(z1_soll) -> [z1_soll_Ausweichen]
  desired trajectory: Parabola/2(z2_soll) -> [z2_soll_Ausweichen]
  [t] -> desired trajectory: Sequence of SP changes/1(t)
  [T] -> desired trajectory: Sequence of SP changes/2(T)
  Demux2/1 -> desired trajectory: Sequence of SP changes/3(z10)
  Demux2/2 -> desired trajectory: Sequence of SP changes/4(z20)
  Constant/1 -> desired trajectory: Sequence of SP changes/5(T_task)
  Constant1/1 -> desired trajectory: Sequence of SP changes/6(x_links)
  Constant2/1 -> desired trajectory: Sequence of SP changes/7(x_rechts)
  Constant3/1 -> desired trajectory: Sequence of SP changes/8(y_oben)
  Constant4/1 -> desired trajectory: Sequence of SP changes/9(y_unten)
  desired trajectory: Sequence of SP changes/1(z1_soll) -> [z1_soll_AP_Wechselfolge]
  desired trajectory: Sequence of SP changes/2(z2_soll) -> [z2_soll_AP_Wechselfolge]

== system Simulation/System model/Kinematisches Modell ==
  Stellgroessen : Inport
  Enable : EnablePort
  Integrator : Integrator  InitialCondition=[param.xW0, 0.0, param.l0, 0.0, 0.0, 0.0]
  "sys_dgl " : MATLAB Function  TreatAsAtomicUnit=on
  Systemzustände : Outport
  wires:
  "sys_dgl "/1(dx) -> Integrator/1
  Integrator/1 -> Systemzustände/1, "sys_dgl "/1(x)
  Stellgroessen/1 -> "sys_dgl "/2(u)

== system Simulation/System model/Referenzmodell ==
  Stellgroessen : Inport
  Enable : EnablePort
  Constant5 : Constant  Value=[0 0 param.xW0 0 param.l0 0]
  Demux : Demux  Outputs=2
  Integrator : Integrator
  Integrator1 : Integrator
  Referenzstrecke : Subsystem
  Selector : Selector  InputPortWidth=6  IndexOptions=Index vector (dialog)  Indices=4  OutputSizes=1
  Selector1 : Selector  InputPortWidth=6  IndexOptions=Index vector (dialog)  Indices=6  OutputSizes=1
  Unterlagerte v-Regelung : Subsystem
  Vorsteuerung Trommel : Subsystem
  Vorsteuerung Wagen : Subsystem
  Zustandsvektor : Selector  InputPortWidth=6  IndexOptions=Index vector (dialog)  Indices=[3 4 5 6 1 2]  OutputSizes=1
  Systemzustaende : Outport
  wires:
  Selector/1 -> Unterlagerte v-Regelung/1(vW)  "vW"
  Selector1/1 -> Unterlagerte v-Regelung/2(vl)  "vL"
  Constant5/1 -> Referenzstrecke/2(xi0)
  Referenzstrecke/1("xi (phi, phip, x, xp, l, lp)") -> Selector/1, Selector1/1, Zustandsvektor/1  "x_truth"
  Zustandsvektor/1 -> Systemzustaende/1  "5"
  Unterlagerte v-Regelung/1(u) -> Referenzstrecke/1("u (F, MT)")
  Stellgroessen/1 -> Demux/1
  Integrator/1 -> Unterlagerte v-Regelung/3(vWDes)
  Integrator1/1 -> Unterlagerte v-Regelung/4(vldes)
  Demux/1 -> Integrator/1, Vorsteuerung Wagen/1(aW)
  Demux/2 -> Vorsteuerung Trommel/1(aS), Integrator1/1
  Vorsteuerung Trommel/1(FF MT) -> Unterlagerte v-Regelung/6(FW_MT)
  Vorsteuerung Wagen/1(FF FW) -> Unterlagerte v-Regelung/5(FW_VS)

== system Simulation/System model1/Kinematisches Modell ==
  Stellgroessen : Inport
  Enable : EnablePort
  Integrator : Integrator  InitialCondition=[param.xW0, 0.0, param.l0, 0.0, 0.0, 0.0]
  "sys_dgl " : MATLAB Function  TreatAsAtomicUnit=on
  Systemzustände : Outport
  wires:
  "sys_dgl "/1(dx) -> Integrator/1
  Integrator/1 -> Systemzustände/1, "sys_dgl "/1(x)
  Stellgroessen/1 -> "sys_dgl "/2(u)

== system Simulation/System model1/Referenzmodell ==
  Stellgroessen : Inport
  Enable : EnablePort
  Constant5 : Constant  Value=[0 0 param.xW0 0 param.l0 0]
  Demux : Demux  Outputs=2
  Integrator : Integrator
  Integrator1 : Integrator
  Referenzstrecke : Subsystem
  Selector : Selector  InputPortWidth=6  IndexOptions=Index vector (dialog)  Indices=4  OutputSizes=1
  Selector1 : Selector  InputPortWidth=6  IndexOptions=Index vector (dialog)  Indices=6  OutputSizes=1
  Unterlagerte v-Regelung : Subsystem
  Vorsteuerung Trommel : Subsystem
  Vorsteuerung Wagen : Subsystem
  Zustandsvektor : Selector  InputPortWidth=6  IndexOptions=Index vector (dialog)  Indices=[3 4 5 6 1 2]  OutputSizes=1
  Systemzustaende : Outport
  wires:
  Selector/1 -> Unterlagerte v-Regelung/1(vW)  "vW"
  Selector1/1 -> Unterlagerte v-Regelung/2(vl)  "vL"
  Constant5/1 -> Referenzstrecke/2(xi0)
  Referenzstrecke/1("xi (phi, phip, x, xp, l, lp)") -> Selector/1, Selector1/1, Zustandsvektor/1  "x_truth"
  Zustandsvektor/1 -> Systemzustaende/1  "5"
  Unterlagerte v-Regelung/1(u) -> Referenzstrecke/1("u (F, MT)")
  Stellgroessen/1 -> Demux/1
  Integrator/1 -> Unterlagerte v-Regelung/3(vWDes)
  Integrator1/1 -> Unterlagerte v-Regelung/4(vldes)
  Demux/1 -> Integrator/1, Vorsteuerung Wagen/1(aW)
  Demux/2 -> Vorsteuerung Trommel/1(aS), Integrator1/1
  Vorsteuerung Trommel/1(FF MT) -> Unterlagerte v-Regelung/6(FW_MT)
  Vorsteuerung Wagen/1(FF FW) -> Unterlagerte v-Regelung/5(FW_VS)

== system Simulation/Flatness-based control/dynamic tracking control/Computation of the flat output ==
  Control input : Inport
  States : Inport  Port=2
  Demux : Demux  Outputs=8
  Demux1 : Demux  Outputs=2
  Derivative : Derivative
  Derivative1 : Derivative
  MATLAB Function : MATLAB Function  TreatAsAtomicUnit=on
  MATLAB Function1 : MATLAB Function  TreatAsAtomicUnit=on
  MATLAB Function2 : MATLAB Function  TreatAsAtomicUnit=on
  Mux : Mux
  Mux1 : Mux
  z1_xLoad : Outport
  z2_yLoad : Outport  Port=2
  wires:
  MATLAB Function/2(z2) -> Mux1/1
  Derivative/1 -> Mux/4
  MATLAB Function2/1(ddz1) -> Mux/3, Derivative/1
  MATLAB Function/1(z1) -> Mux/1
  Demux/2 -> MATLAB Function1/1(x2)
  Demux/6 -> MATLAB Function2/3(x6), MATLAB Function1/5(x6)
  MATLAB Function2/2(ddz2) -> Mux1/3, Derivative1/1
  Control input/1 -> Demux1/1
  MATLAB Function1/2(dz2) -> Mux1/2
  Demux/5 -> MATLAB Function/3(x5), MATLAB Function2/2(x5), MATLAB Function1/4(x5)
  Demux/1 -> MATLAB Function/1(x1)
  States/1 -> Demux/1
  Demux/3 -> MATLAB Function2/1(x3), MATLAB Function1/2(x3), MATLAB Function/2(x3)
  Demux/4 -> MATLAB Function1/3(x4)
  MATLAB Function1/1(dz1) -> Mux/2
  Derivative1/1 -> Mux1/4
  Mux/1 -> z1_xLoad/1
  Mux1/1 -> z2_yLoad/1
  Demux1/1 -> MATLAB Function2/4(u1)
  Demux1/2 -> MATLAB Function2/5(u2)

== system Simulation/Flatness-based control/dynamic tracking control/System extension ==
  u_extended : Inport
  x_real : Inport  Port=2
  Demux : Demux  Outputs=6
  Demux1 : Demux  Outputs=2
  Integrator : Integrator
  Integrator1 : Integrator
  MATLAB Function3 : MATLAB Function  TreatAsAtomicUnit=on
  Mux : Mux  Inputs=8
  u2_real : Outport
  x_extended : Outport  Port=2
  wires:
  u_extended/1 -> Demux1/1
  x_real/1 -> Demux/1
  Mux/1 -> x_extended/1
  Demux/1 -> Mux/1
  Demux1/1 -> MATLAB Function3/5(u1_ext), Mux/2
  Demux/3 -> Mux/3, MATLAB Function3/2(x3)
  MATLAB Function3/1(u2_real) -> Mux/4, u2_real/1
  Demux/5 -> MATLAB Function3/3(x5), Mux/5
  Demux/6 -> Mux/6, MATLAB Function3/4(x6)
  Demux1/2 -> Integrator/1
  Integrator/1 -> Mux/8, Integrator1/1  "x2_ext"
  Integrator1/1 -> Mux/7, MATLAB Function3/1(x1_ext)  "x1_ext"

== system Simulation/Flatness-based control/dynamic tracking control/Tracking controller ==
  z1_xLoad : Inport
  z2_yLoad : Inport  Port=2
  z1_d_xLoad : Inport  Port=3
  z2_d_yLoad : Inport  Port=4
  Constant : Constant  Value=[param.pX01 param.pX02 param.pX03 param.pX04]
  Constant1 : Constant  Value=[param.pY01_DYN param.pY02_DYN param.pY03_DYN param.pY04_DYN]
  Demux : Demux
  Demux1 : Demux
  MATLAB Function : MATLAB Function  TreatAsAtomicUnit=on
  Tracking controller v1 for xLoad : Subsystem
  Tracking controller v2 for yLoad : Subsystem
  u1_aCart : Outport
  u2_aRope : Outport  Port=2
  wires:
  Constant1/1 -> Tracking controller v2 for yLoad/3(Koeffizienten2)
  Constant/1 -> Tracking controller v1 for xLoad/3(Koeffizienten1)
  z2_d_yLoad/1 -> Tracking controller v2 for yLoad/1(z2_soll)
  z1_d_xLoad/1 -> Tracking controller v1 for xLoad/1(z1_soll)
  z1_xLoad/1 -> Demux/1, Tracking controller v1 for xLoad/2(z1_ist)
  MATLAB Function/2(u2) -> u2_aRope/1
  Demux1/1 -> MATLAB Function/4(z2)
  Demux/4 -> MATLAB Function/2(dddz1)
  z2_yLoad/1 -> Demux1/1, Tracking controller v2 for yLoad/2(z2_ist)
  Demux1/2 -> MATLAB Function/5(dz2)
  Tracking controller v1 for xLoad/1(v1) -> MATLAB Function/3(v1)
  MATLAB Function/1(u1) -> u1_aCart/1
  Demux/3 -> MATLAB Function/1(ddz1)
  Tracking controller v2 for yLoad/1(v2) -> MATLAB Function/8(v2)
  Demux1/3 -> MATLAB Function/6(ddz2)
  Demux1/4 -> MATLAB Function/7(dddz2)

== system Simulation/Flatness-based control/quasistatic tracking control/Computation of the flat output ==
  Control input : Inport
  States : Inport  Port=2
  Demux : Demux  Outputs=6
  Demux1 : Demux  Outputs=2
  Derivative : Derivative
  Derivative1 : Derivative
  MATLAB Function : MATLAB Function  TreatAsAtomicUnit=on
  MATLAB Function1 : MATLAB Function  TreatAsAtomicUnit=on
  MATLAB Function2 : MATLAB Function  TreatAsAtomicUnit=on
  Mux : Mux
  Mux1 : Mux
  z1_xLoad : Outport
  z2_yLoad : Outport  Port=2
  wires:
  States/1 -> Demux/1
  Demux/1 -> MATLAB Function/1(x1)
  Demux/3 -> MATLAB Function2/1(x3), MATLAB Function1/2(x3), MATLAB Function/2(x3)
  Demux/5 -> MATLAB Function/3(x5), MATLAB Function2/2(x5), MATLAB Function1/4(x5)
  Control input/1 -> Demux1/1
  Mux1/1 -> z2_yLoad/1
  Mux/1 -> z1_xLoad/1
  Demux/2 -> MATLAB Function1/1(x2)
  Demux/4 -> MATLAB Function1/3(x4)
  Demux/6 -> MATLAB Function2/3(x6), MATLAB Function1/5(x6)
  Demux1/1 -> MATLAB Function2/4(u1)
  Demux1/2 -> MATLAB Function2/5(u2)
  MATLAB Function2/1(ddz1) -> Mux/3, Derivative/1
  MATLAB Function2/2(ddz2) -> Mux1/3, Derivative1/1
  Derivative/1 -> Mux/4
  Derivative1/1 -> Mux1/4
  MATLAB Function1/2(dz2) -> Mux1/2
  MATLAB Function/2(z2) -> Mux1/1
  MATLAB Function/1(z1) -> Mux/1
  MATLAB Function1/1(dz1) -> Mux/2

== system Simulation/Flatness-based control/quasistatic tracking control/Tracking controller ==
  z1_xLoad : Inport
  z2_yLoad : Inport  Port=2
  z1_d_xLoad : Inport  Port=3
  z2_d_yLoad : Inport  Port=4
  Constant : Constant  Value=[param.pX01 param.pX02 param.pX03 param.pX04]
  Constant1 : Constant  Value=[param.pY01_QS param.pY02_QS]
  Demux : Demux
  Demux1 : Demux
  MATLAB Function : MATLAB Function  TreatAsAtomicUnit=on
  Tracking controller v1 for xLoad : Subsystem
  Tracking controller v2 for yLoad : Subsystem
  u1_aCart : Outport
  u2_aRope : Outport  Port=2
  wires:
  Constant1/1 -> Tracking controller v2 for yLoad/3(Koeffizienten2)
  Constant/1 -> Tracking controller v1 for xLoad/3(Koeffizienten1)
  z2_yLoad/1 -> Demux1/1, Tracking controller v2 for yLoad/2(z2_ist)
  z2_d_yLoad/1 -> Tracking controller v2 for yLoad/1(z2_soll)
  z1_xLoad/1 -> Demux/1, Tracking controller v1 for xLoad/2(z1_ist)
  z1_d_xLoad/1 -> Tracking controller v1 for xLoad/1(z1_soll)
  MATLAB Function/1(u1) -> u1_aCart/1
  MATLAB Function/2(u2) -> u2_aRope/1
  Tracking controller v2 for yLoad/3(ddv2) -> MATLAB Function/8(ddv2)
  Tracking controller v2 for yLoad/2(dv2) -> MATLAB Function/7(dv2)
  Tracking controller v2 for yLoad/1(v2) -> MATLAB Function/6(v2)
  Tracking controller v1 for xLoad/1(v1) -> MATLAB Function/3(v1)
  Demux/4 -> MATLAB Function/2(dddz1)
  Demux/3 -> MATLAB Function/1(ddz1)
  Demux1/1 -> MATLAB Function/4(z2)
  Demux1/2 -> MATLAB Function/5(dz2)
